simulink model "motor_model"  (R2018a)
settings: Solver=VariableStepAuto  StartTime=0.0  StopTime=2  RelTol=1e-3
libraries: powerlib x14, powerlib_meascontrol x1, powerlib_extras x1
settings Model: Creator=HP  LastModifiedBy=HP

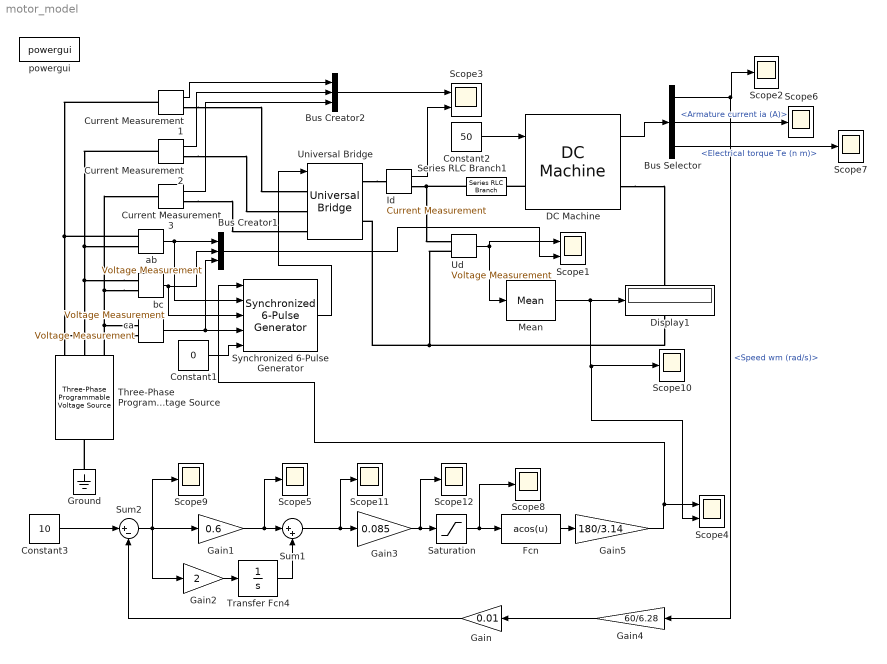
== system motor_model ==
  Bus Creator1 : BusCreator  Inputs=3
  Bus Creator2 : BusCreator  Inputs=3
  Bus Selector : BusSelector  OutputSignals=Speed wm (rad/s),Armature current ia (A),Electrical torque Te (n m)
  Constant1 : Constant  Value=0
  Constant2 : Constant  Value=50
  Constant3 : Constant  Value=10
  Current Measurement1 : powerlib/Measurements/Current Measurement  PhasorSimulation=off  OutputType=Complex  PSBequivalent=0
  Current Measurement2 : powerlib/Measurements/Current Measurement  PhasorSimulation=off  OutputType=Complex  PSBequivalent=0
  Current Measurement3 : powerlib/Measurements/Current Measurement  PhasorSimulation=off  OutputType=Complex  PSBequivalent=0
  DC Machine : powerlib/Machines/DC Machine  PresetModel=No  MechanicalLoad=Torque TL  FieldType=Permanent magnet  ShowDetailedParameters=on  MeasurementBus=off  RLa="[ 1  0.00167]"  RLf="[ 240  120]"  Laf=1.8  MachineConstant=Back-emf constant (V/rpm)  Ke=0.192  Kt=1.8  J=1  Bm=0  Tf=0  w0=0  Ifinit=1  TsPowergui=0  TsBlock=-1
  Display1 : Display
  Fcn : Fcn  Expr=acos(u)
  Gain : Gain  Gain=0.01
  Gain1 : Gain  Gain=0.6
  Gain2 : Gain  Gain=2
  Gain3 : Gain  Gain=0.085
  Gain4 : Gain  Gain=60/6.28
  Gain5 : Gain  Gain=180/3.14
  Ground : powerlib/Elements/Ground  LConnTagsString=a
  "Id " : powerlib/Measurements/Current Measurement  PhasorSimulation=off  OutputType=Complex  PSBequivalent=0
  Mean : powerlib_meascontrol/Measurements/Mean  Freq=50  Vinit=0  Ts=0
  Saturation : Saturate  UpperLimit=1  LowerLimit=-1
  Scope1 : Scope  NumInputPorts=2
  Scope{2,5..12} (9 alike) : Scope
  Scope3 : Scope  NumInputPorts=2
  Scope4 : Scope  NumInputPorts=2
  Series RLC Branch1 : powerlib/Elements/Series RLC Branch  LConnTagsString=__new0  RConnTagsString=__new0  BranchType=L  Resistance=0  Inductance=0.02  SetiL0=off  InitialCurrent=0  Capacitance=1.0  Setx0=off  InitialVoltage=0  Measurements=None
  Sum1 : Sum  Inputs=|++
  Sum2 : Sum  Inputs=|+-
  Synchronized 6-Pulse Generator : powerlib_extras/Control  Blocks/Synchronized 6-Pulse Generator  freq=50  pwidth=10  Double_Pulse=off
  Three-Phase Programmable Voltage Source : powerlib/Electrical Sources/Three-Phase Programmable Voltage Source  PositiveSequence="[380  0 50]"  VariationEntity=None  VariationType=Step  VariationTypeAlt=Step  VariationStep=0.5  VariationRate=10  VariationMagnitude=0.3  VariationFrequency=2  VariationTiming=[1 2]  VariationPhaseA=off  Amplitudes=[1 0.8 1.2 1.0]  TimeValues=[0 0.1 0.15 0.2]  HarmonicGeneration=off  HarmonicA=[3 0.2 -25 0]  HarmonicB=[2 0.15 35 2]  Timing="[0.05  3]"  BusType=swing  Pref=0  Qref=0  Qmin=-inf  Qmax=inf
  Transfer Fcn4 : TransferFcn  Denominator=[1 0]
  "Ud " : powerlib/Measurements/Voltage Measurement  PhasorSimulation=off  OutputType=Complex  PSBequivalent=0
  Universal Bridge : powerlib/Power Electronics/Universal Bridge  Arms=3  SnubberResistance=47  SnubberCapacitance=1e-5  Device=Thyristors  Ron=0  Lon=0  ForwardVoltages="[  0  0  ]"  ForwardVoltage=0  GTOparameters=[ 10e-6 , 20e-6 ]  IGBTparameters=[ 1e-6 , 2e-6 ]  Measurements=None  Measurements_2=None  converterType=Rectifier
  ab : powerlib/Measurements/Voltage Measurement  PhasorSimulation=off  OutputType=Complex  PSBequivalent=0
  "bc " : powerlib/Measurements/Voltage Measurement  PhasorSimulation=off  OutputType=Complex  PSBequivalent=0
  "ca " : powerlib/Measurements/Voltage Measurement  PhasorSimulation=off  OutputType=Complex  PSBequivalent=0
  powergui : powerlib/powergui  SimulationMode=Continuous  SampleTime=50e-7  frequency=60  Iterations=50  frequencyindice=0  Pbase=100e6  ErrMax=1e-4  UnitsV=kV  UnitsW=MW  buscounter=0  FunctionMessages=off  echomessages=off  EnableUseOfTLC=off  CurrentSourceSwitches=off  DisableSnubberDevices=off  DisableRonSwitches=off  DisableVfSwitches=off  DisplayEquations=off  SolverType=Tustin/Backward Euler (TBE)  Interpol=off  ExternalGateDelay=off  methode=off  Ts=100  x0status=blocks  SPID=off  SwTol=0  HookPort=off  RestoreLinks=warning  ResistiveCurrentMeasurement=off  Frange=[0:2:500]  Ylog=off  Xlog=on  ShowGrid=off  save=off  variable=ZData  structure=ScopeData6  ZoomFFT=off  StartTime=0.6  cycles=3  DisplayStyle=1  fundamental=50  FreqAxis=off  MaxFrequency=1000  frequencyindicesteady=1  RmsSteady=1  display=off
  wires:
  Current Measurement2/1 -> Bus Creator2/2
  Synchronized 6-Pulse Generator/1 -> Universal Bridge/1
  "Ud "/1 -> Scope1/1, Mean/1
  "ca "/1 -> Bus Creator1/3, Synchronized 6-Pulse Generator/4
  Current Measurement3/1 -> Bus Creator2/3
  "bc "/1 -> Bus Creator1/2, Synchronized 6-Pulse Generator/3
  ab/1 -> Bus Creator1/1, Synchronized 6-Pulse Generator/2
  Constant1/1 -> Synchronized 6-Pulse Generator/5
  Current Measurement1/1 -> Bus Creator2/1
  "Id "/1 -> Scope3/2
  Fcn/1 -> Gain5/1
  DC Machine/1 -> Bus Selector/1
  Mean/1 -> Scope4/2, Scope10/1, Display1/1
  Constant2/1 -> DC Machine/1
  Bus Selector/1 -> Gain4/1, Scope2/1  "<Speed wm (rad/s)>"
  Bus Selector/2 -> Scope6/1  "<Armature current ia (A)>"
  Bus Selector/3 -> Scope7/1  "<Electrical torque Te (n m)>"
  Constant3/1 -> Sum2/1
  Gain2/1 -> Transfer Fcn4/1
  Transfer Fcn4/1 -> Sum1/2
  Sum2/1 -> Gain2/1, Scope9/1, Gain1/1
  Gain4/1 -> Gain/1
  Saturation/1 -> Scope8/1, Fcn/1
  Sum1/1 -> Scope11/1, Gain3/1
  Gain3/1 -> Scope12/1, Saturation/1
  Gain5/1 -> Synchronized 6-Pulse Generator/1, Scope4/1
  Gain/1 -> Sum2/2
  Bus Creator2/1 -> Scope3/1
  Bus Creator1/1 -> Scope1/2
  Gain1/1 -> Scope5/1, Sum1/1
  connections:
  Universal Bridge/RConn1 -- "Id "/LConn1
  ab/LConn1 -- Current Measurement1/LConn1 -- "ca "/LConn2 -- Three-Phase Programmable Voltage Source/RConn1
  "Ud "/LConn2 -- DC Machine/RConn1 -- Universal Bridge/RConn2
  Current Measurement1/RConn1 -- Universal Bridge/LConn1
  "bc "/LConn2 -- Three-Phase Programmable Voltage Source/RConn3 -- "ca "/LConn1 -- Current Measurement3/LConn1
  Current Measurement2/RConn1 -- Universal Bridge/LConn2
  "bc "/LConn1 -- Current Measurement2/LConn1 -- ab/LConn2 -- Three-Phase Programmable Voltage Source/RConn2
  Current Measurement3/RConn1 -- Universal Bridge/LConn3
  Ground/LConn1 -- Three-Phase Programmable Voltage Source/LConn1
  DC Machine/LConn1 -- Series RLC Branch1/LConn1
  "Id "/RConn1 -- "Ud "/LConn1 -- Series RLC Branch1/RConn1
